simulink model "zad6"  (R2021a)
settings: Solver=VariableStepAuto  StartTime=0.0  StopTime=5  RelTol=1e-3
values from neighbouring files (symbols this model uses):
  k1 = k(1,1)    [liczenie_k.m]    (also in skrypt_k_i_l.m; zad4.m; zad_dod.m = K(1))
  k2 = k(1,2)    [liczenie_k.m]    (also in skrypt_k_i_l.m; zad4.m; zad_dod.m = K(2))
  k3 = k(1,3)    [liczenie_k.m]    (also in skrypt_k_i_l.m; zad4.m; zad_dod.m = K(3))
  L1 = L(1)    [liczenie_l_num.m]    (also in skrypt_k_i_l.m)
  L2 = L(2)    [liczenie_l_num.m]    (also in skrypt_k_i_l.m)
  L3 = L(3)    [liczenie_l_num.m]    (also in skrypt_k_i_l.m)
settings Model: Creator=ADMIN  LastModifiedBy=ADMIN

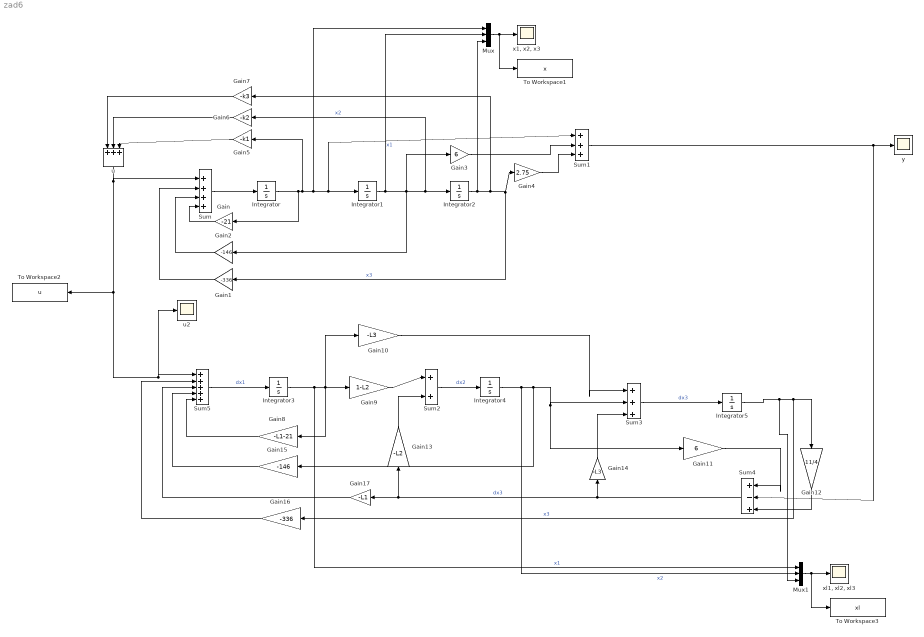
== system zad6 ==
  Gain : Gain  Gain=-21
  Gain1 : Gain  Gain=-336
  Gain10 : Gain  Gain=-L3
  Gain11 : Gain  Gain=6
  Gain12 : Gain  Gain=11/4
  Gain13 : Gain  Gain=-L2
  Gain14 : Gain  Gain=-L3
  Gain15 : Gain  Gain=-146
  Gain16 : Gain  Gain=-336
  Gain17 : Gain  Gain=-L1
  Gain2 : Gain  Gain=-146
  Gain3 : Gain  Gain=6
  Gain4 : Gain  Gain=2.75
  Gain5 : Gain  Gain=-k1
  Gain6 : Gain  Gain=-k2
  Gain7 : Gain  Gain=-k3
  Gain8 : Gain  Gain=-L1-21
  Gain9 : Gain  Gain=1-L2
  Integrator : Integrator  InitialCondition=1
  Integrator1 : Integrator  InitialCondition=2
  Integrator2 : Integrator  InitialCondition=4
  Integrator3 : Integrator
  Integrator4 : Integrator
  Integrator5 : Integrator
  Mux : Mux  Inputs=3
  Mux1 : Mux  Inputs=3
  Sum : Sum  Inputs=|++++
  Sum1 : Sum  Inputs=|+++
  Sum2 : Sum  Inputs=|++
  Sum3 : Sum  Inputs=|+++
  Sum4 : Sum  Inputs=|+-+
  Sum5 : Sum  Inputs=|+++++
  To Workspace1 : ToWorkspace  VariableName=x  SaveFormat=Structure With Time  SampleTime=-1
  To Workspace2 : ToWorkspace  VariableName=u  SaveFormat=Structure With Time  SampleTime=-1
  To Workspace3 : ToWorkspace  VariableName=xl  SaveFormat=Structure With Time  SampleTime=-1
  u : Sum  Inputs=+++
  u2 : Scope
  "x1, x2, x3" : Scope
  "xl1, xl2, xl3" : Scope
  y : Scope
  wires:
  Gain4/1 -> Sum1/3
  Gain5/1 -> u/3
  Integrator2/1 -> Mux/3, Gain7/1, Gain4/1, Gain1/1  "x3"
  Gain6/1 -> u/2
  Gain/1 -> Sum/4
  Gain2/1 -> Sum/3
  Integrator/1 -> Gain5/1, Mux/1, Sum1/1, Integrator1/1, Gain/1  "x1"
  Integrator1/1 -> Mux/2, Gain3/1, Gain2/1, Gain6/1, Integrator2/1  "x2"
  Sum/1 -> Integrator/1
  Gain3/1 -> Sum1/2
  Gain7/1 -> u/1
  Mux/1 -> To Workspace1/1, "x1, x2, x3"/1
  Gain1/1 -> Sum/2
  Mux1/1 -> To Workspace3/1, "xl1, xl2, xl3"/1
  Gain14/1 -> Sum3/3
  Gain17/1 -> Sum5/3
  Gain13/1 -> Sum2/2
  Gain8/1 -> Sum5/5
  Sum1/1 -> Sum4/2, y/1
  Integrator3/1 -> Mux1/1, Gain10/1, Gain9/1, Gain8/1  "x1"
  Sum4/1 -> Gain14/1, Gain17/1, Gain13/1  "dx3"
  Sum2/1 -> Integrator4/1  "dx2"
  Integrator5/1 -> Mux1/3, Gain16/1, Gain12/1  "x3"
  Sum3/1 -> Integrator5/1  "dx3"
  Gain9/1 -> Sum2/1
  Integrator4/1 -> Mux1/2, Gain15/1, Sum3/2, Gain11/1  "x2"
  Sum5/1 -> Integrator3/1  "dx1"
  Gain15/1 -> Sum5/4
  Gain16/1 -> Sum5/2
  u/1 -> u2/1, Sum5/1, To Workspace2/1, Sum/1
  Gain11/1 -> Sum4/1
  Gain12/1 -> Sum4/3
  Gain10/1 -> Sum3/1
